simulink model "E2_1"  (R2022a)
settings: Solver=VariableStepAuto  StartTime=0.0  StopTime=10.0  RelTol=1e-3
settings Model: Creator=Reza  LastModifiedBy=Reza

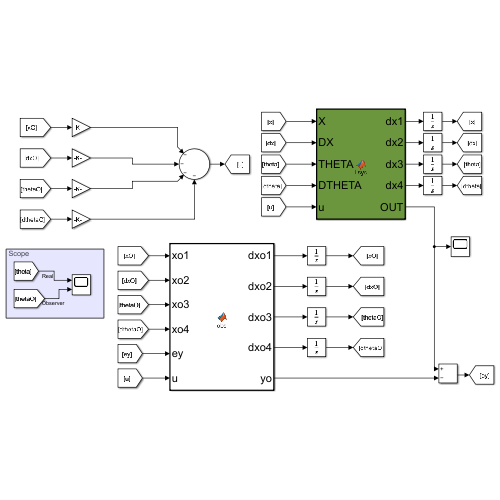
[thumbnail: Simulink's stored preview of the top-level diagram]
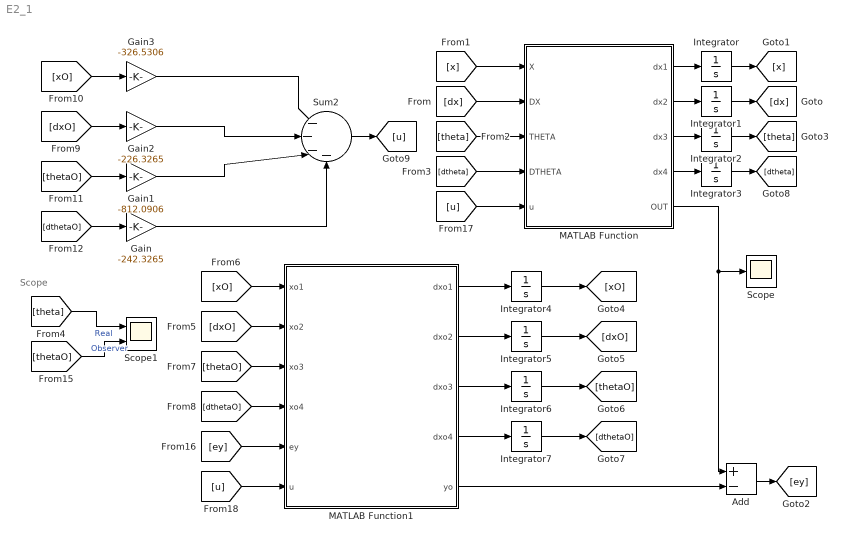
== system E2_1 ==
  note: Scope
  Add : Sum  Inputs=+-
  Gain : Gain  Gain=-242.3265
  Gain1 : Gain  Gain=-812.0906
  Gain2 : Gain  Gain=-226.3265
  Gain3 : Gain  Gain=-326.5306
  Integrator{,1,3..7} (7 alike) : Integrator
  Integrator2 : Integrator  InitialCondition=10*pi/180
  MATLAB Function : MATLAB Function  TreatAsAtomicUnit=on
  MATLAB Function1 : MATLAB Function  TreatAsAtomicUnit=on
  Scope : Scope
  Scope1 : Scope  NumInputPorts=2
  Sum2 : Sum  Inputs=|----
  wires:
  Sum2/1 -> [u]
  Integrator3/1 -> [dtheta]
  [thetaO] -> Scope1/2  "Observer"
  [xO] -> Gain3/1
  [dthetaO] -> Gain/1
  Integrator4/1 -> [xO]
  Integrator7/1 -> [dthetaO]
  Integrator5/1 -> [dxO]
  [x] -> MATLAB Function/1(X)
  [theta] -> MATLAB Function/3(THETA)
  [xO] -> MATLAB Function1/1(xo1)
  [theta] -> Scope1/1  "Real"
  [dthetaO] -> MATLAB Function1/4(xo4)
  [dxO] -> MATLAB Function1/2(xo2)
  Add/1 -> [ey]
  [thetaO] -> MATLAB Function1/3(xo3)
  [dx] -> MATLAB Function/2(DX)
  Integrator1/1 -> [dx]
  [dtheta] -> MATLAB Function/4(DTHETA)
  [ey] -> MATLAB Function1/5(ey)
  MATLAB Function1/4(dxo4) -> Integrator7/1
  MATLAB Function1/5(yo) -> Add/2
  Gain2/1 -> Sum2/2
  MATLAB Function1/2(dxo2) -> Integrator5/1
  Gain3/1 -> Sum2/1
  Integrator6/1 -> [thetaO]
  Gain/1 -> Sum2/4
  Gain1/1 -> Sum2/3
  [u] -> MATLAB Function1/6(u)
  MATLAB Function/2(dx2) -> Integrator1/1
  MATLAB Function1/3(dxo3) -> Integrator6/1
  Integrator2/1 -> [theta]
  MATLAB Function1/1(dxo1) -> Integrator4/1
  MATLAB Function/4(dx4) -> Integrator3/1
  [u] -> MATLAB Function/5(u)
  MATLAB Function/3(dx3) -> Integrator2/1
  Integrator/1 -> [x]
  MATLAB Function/1(dx1) -> Integrator/1
  [thetaO] -> Gain1/1
  [dxO] -> Gain2/1
  MATLAB Function/5(OUT) -> Add/1, Scope/1

== matlab function E2_1/MATLAB Function1 ==
  data: xo1 input; xo2 input; xo3 input; xo4 input; ey input; u input; dxo1 output; dxo2 output; dxo3 output; dxo4 output; yo output
function [dxo1,dxo2,dxo3,dxo4,yo] = obs(xo1,xo2,xo3,xo4,ey,u)


m = 0.1 ;
M = 1.0 ;
L = 1.0 ;
g = 10 ;
k = 1 ;
R = 100 ;
r = 0.02 ;

A = [ 0 ,           1           ,         0        , 0 ;
      0 ,   (-k^2/(M*R*r^2))    ,       -m*g/M     , 0 ;
      0 ,            0          ,         0        , 1 ;
      0 ,   (k^2/(M*R*r^2*L))   ,  ((M+m)*g/(M*L)) , 0 ] ;

B = [0 ; k/(M*R*r) ; 0 ;  -k/(M*R*r*L) ] ;

C = [ 1 , 0 , 0 , 0 ] ;

D = 0 ;

xo = [xo1;xo2;xo3;xo4];
L = [-11.9350;394.5103;-452.0058;-1993.6188];
dxo = A*xo+B*u+L*ey;
dxo1 = dxo(1);
dxo2 = dxo(2);
dxo3 = dxo(3);
dxo4 = dxo(4);
yo = C*xo+D*u;

== matlab function E2_1/MATLAB Function ==
  data: X input; DX input; THETA input; DTHETA input; dx1 output; dx2 output; dx3 output; dx4 output; u input; OUT output
function [dx1,dx2,dx3,dx4,OUT] = Lsys(X,DX,THETA,DTHETA,u)


m = 0.1 ;
M = 1.0 ;
L = 1.0 ;
g = 10 ;
k = 1 ;
R = 100 ;
r = 0.02 ;

A = [ 0 ,           1           ,         0        , 0 ;
      0 ,   (-k^2/(M*R*r^2))    ,       -m*g/M     , 0 ;
      0 ,            0          ,         0        , 1 ;
      0 ,   (k^2/(M*R*r^2*L))   ,  ((M+m)*g/(M*L)) , 0 ] ;

B = [0 ; k/(M*R*r) ; 0 ;  -k/(M*R*r*L) ] ;

C = [ 1 , 0 , 0 , 0 ] ;

D = 0 ;

x = [X;DX;THETA;DTHETA];
dx = A*x+B*u;
dx1 = dx(1);
dx2 = dx(2);
dx3 = dx(3);
dx4 = dx(4);
OUT = C*x+D*u;
